simulink model "Reduce_Block_Diagram_Manual_1"  (R2024a)
settings: Solver=VariableStepAuto  StartTime=0.0  StopTime=10.0  RelTol=1e-3
values from neighbouring files (symbols this model uses):
  G1_den = [1 0 0]    [Reduce_Block_Diagram_1.m]
  G1_num = [1]    [Reduce_Block_Diagram_1.m]    (also in Reduce_Block_Diagram_2.m)
  G2_den = [1 1]    [Reduce_Block_Diagram_1.m]    (also in Reduce_Block_Diagram_2.m)
  G2_num = [1]    [Reduce_Block_Diagram_1.m]    (also in Reduce_Block_Diagram_2.m)
  G3_den = [1 0]    [Reduce_Block_Diagram_1.m]    (also in Reduce_Block_Diagram_2.m)
  G3_num = [1]    [Reduce_Block_Diagram_1.m]    (also in Reduce_Block_Diagram_2.m)
  H1_den = [1 0]    [Reduce_Block_Diagram_1.m]
  H1_num = [1]    [Reduce_Block_Diagram_1.m]
  H2_den = [1 -1]    [Reduce_Block_Diagram_1.m]
  H2_num = [1]    [Reduce_Block_Diagram_1.m]
  H3_den = [1 -2]    [Reduce_Block_Diagram_1.m]
  H3_num = [1]    [Reduce_Block_Diagram_1.m]
undefined symbols (not defined in the file or in its folder): G21_den, G21_num, G23_den, G23_num, TF2_den, TF2_num, TF3_den, TF3_num, TF4_den, TF4_num, TF_den, TF_num

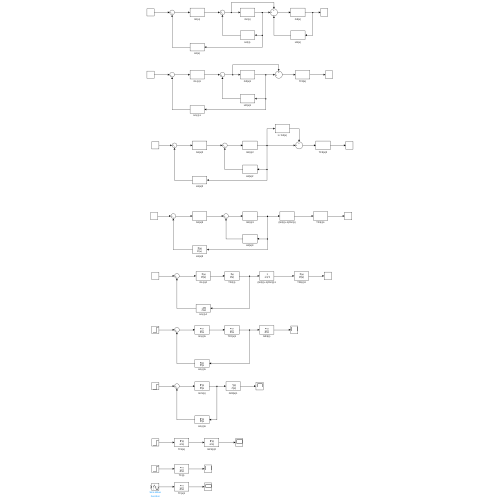
[thumbnail: Simulink's stored preview of the top-level diagram]
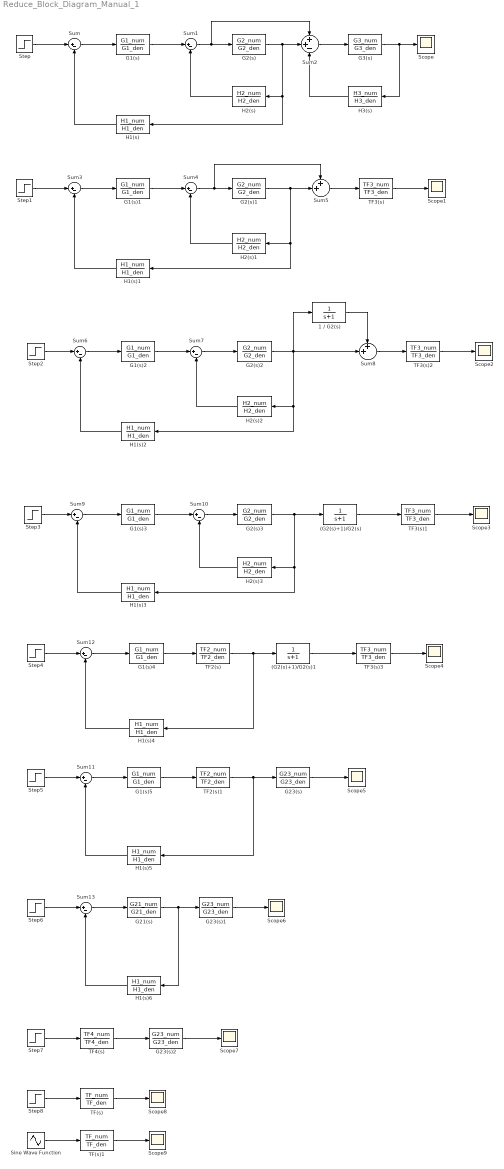
== system Reduce_Block_Diagram_Manual_1 ==
  (G2(s)+1)/G2(s) : TransferFcn  Denominator=[1 1]
  (G2(s)+1)/G2(s)1 : TransferFcn  Denominator=[1 1]
  1 / G2(s) : TransferFcn  Denominator=[1 1]
  G1(s){,1..5} (6 alike) : TransferFcn  Numerator=G1_num  Denominator=G1_den
  G2(s){,1..3} (4 alike) : TransferFcn  Numerator=G2_num  Denominator=G2_den
  G21(s) : TransferFcn  Numerator=G21_num  Denominator=G21_den
  G23(s) : TransferFcn  Numerator=G23_num  Denominator=G23_den
  G23(s)1 : TransferFcn  Numerator=G23_num  Denominator=G23_den
  G23(s)2 : TransferFcn  Numerator=G23_num  Denominator=G23_den
  G3(s) : TransferFcn  Numerator=G3_num  Denominator=G3_den
  H1(s){,1..6} (7 alike) : TransferFcn  Numerator=H1_num  Denominator=H1_den
  H2(s){,1..3} (4 alike) : TransferFcn  Numerator=H2_num  Denominator=H2_den
  H3(s) : TransferFcn  Numerator=H3_num  Denominator=H3_den
  Scope{,1..9} (10 alike) : Scope
  Sine Wave Function : Sin  TimeSource=Use external signal  SampleTime=0
  Step{,1..8} (9 alike) : Step  SampleTime=0
  Sum{,1,3..4,6..7,9..13} (11 alike) : Sum  Inputs=|+-
  Sum2 : Sum  Inputs=++-
  Sum5 : Sum  Inputs=++|
  Sum8 : Sum  Inputs=++|
  TF(s) : TransferFcn  Numerator=TF_num  Denominator=TF_den
  TF(s)1 : TransferFcn  Numerator=TF_num  Denominator=TF_den
  TF2(s) : TransferFcn  Numerator=TF2_num  Denominator=TF2_den
  TF2(s)1 : TransferFcn  Numerator=TF2_num  Denominator=TF2_den
  TF3(s){,1..3} (4 alike) : TransferFcn  Numerator=TF3_num  Denominator=TF3_den
  TF4(s) : TransferFcn  Numerator=TF4_num  Denominator=TF4_den
  wires:
  Step/1 -> Sum/1
  Sum/1 -> G1(s)/1
  G3(s)/1 -> H3(s)/1, Scope/1
  H1(s)/1 -> Sum/2
  G1(s)/1 -> Sum1/1
  H2(s)/1 -> Sum1/2
  Sum1/1 -> Sum2/1, G2(s)/1
  Sum2/1 -> G3(s)/1
  G2(s)/1 -> H1(s)/1, H2(s)/1, Sum2/2
  H3(s)/1 -> Sum2/3
  Sum4/1 -> G2(s)1/1, Sum5/1
  G1(s)1/1 -> Sum4/1
  Sum5/1 -> TF3(s)/1
  Step1/1 -> Sum3/1
  TF3(s)/1 -> Scope1/1
  Sum3/1 -> G1(s)1/1
  TF3(s)2/1 -> Scope2/1
  Sum7/1 -> G2(s)2/1
  Sum6/1 -> G1(s)2/1
  G2(s)2/1 -> H1(s)2/1, H2(s)2/1, 1 / G2(s)/1, Sum8/2
  1 / G2(s)/1 -> Sum8/1
  Sum8/1 -> TF3(s)2/1
  G1(s)2/1 -> Sum7/1
  Step2/1 -> Sum6/1
  Sum10/1 -> G2(s)3/1
  H1(s)3/1 -> Sum9/2
  Step3/1 -> Sum9/1
  G1(s)3/1 -> Sum10/1
  Sum9/1 -> G1(s)3/1
  H2(s)3/1 -> Sum10/2
  TF3(s)1/1 -> Scope3/1
  (G2(s)+1)/G2(s)/1 -> TF3(s)1/1
  G2(s)3/1 -> H2(s)3/1, H1(s)3/1, (G2(s)+1)/G2(s)/1
  TF2(s)/1 -> H1(s)4/1, (G2(s)+1)/G2(s)1/1
  (G2(s)+1)/G2(s)1/1 -> TF3(s)3/1
  G1(s)4/1 -> TF2(s)/1
  Sum12/1 -> G1(s)4/1
  H1(s)4/1 -> Sum12/2
  Step4/1 -> Sum12/1
  TF3(s)3/1 -> Scope4/1
  Step5/1 -> Sum11/1
  H1(s)5/1 -> Sum11/2
  G23(s)/1 -> Scope5/1
  TF2(s)1/1 -> H1(s)5/1, G23(s)/1
  Sum11/1 -> G1(s)5/1
  G1(s)5/1 -> TF2(s)1/1
  Step6/1 -> Sum13/1
  G21(s)/1 -> H1(s)6/1, G23(s)1/1
  G23(s)1/1 -> Scope6/1
  H1(s)6/1 -> Sum13/2
  Sum13/1 -> G21(s)/1
  Step7/1 -> TF4(s)/1
  G23(s)2/1 -> Scope7/1
  TF4(s)/1 -> G23(s)2/1
  TF(s)/1 -> Scope8/1
  Step8/1 -> TF(s)/1
  H1(s)1/1 -> Sum3/2
  G2(s)1/1 -> H1(s)1/1, H2(s)1/1, Sum5/2
  H2(s)1/1 -> Sum4/2
  H1(s)2/1 -> Sum6/2
  H2(s)2/1 -> Sum7/2
  TF(s)1/1 -> Scope9/1
  Sine Wave Function/1 -> TF(s)1/1
